simulink model "MMR_IntegratedSimulation_FUZZYTEST"  (R2013a)
settings: Solver=ode3  StartTime=0.0  StopTime=Tstop  FixedStep=1e-2  RelTol=1e-3
values from neighbouring files (symbols this model uses):
  B = 0.0141    [parameters.m]
  Experiment = 2    [parameters.m]
  J = 0.0294    [parameters.m]
  Ke = 0.65    [parameters.m]
  Kt = 0.65    [parameters.m]
  L = 0.04    [parameters.m]
  Len = dis    (= 0)    [calc_len.m]    (also in parameters.m = 0.2)
  r = round(t/step + 1)    [TrajGen_MMR_FUZZYTEST.m]    (also in parameters.m = 0.045)
  R = 3.07    [parameters.m]
  R1_phi = 0.0    (= 0)    [parameters.m]
  R1_xi = 2.0    (= 2)    [parameters.m]
  R1_yi = 0.9    [parameters.m]
  R2_phi = 0.0    (= 0)    [parameters.m]
  R2_xi = -1.0    (= -1)    [parameters.m]
  R2_yi = 4.0    (= 4)    [parameters.m]
  R3_phi = 0.0    (= 0)    [parameters.m]
  R3_xi = 2.0    (= 2)    [parameters.m]
  R3_yi = -1.2    [parameters.m]
  Tstop = 210    [parameters.m]
libraries: simulink x9, fuzblock x6, dsparch4 x3
(part 1 of 2)
settings Model: Creator=Hussain  LastModifiedBy=Hussain Aftab
settings DataIOCC: SignalLoggingSaveFormat=ModelDataLogs
settings DebuggingCC: FcnCallInpInsideContextMsg=EnableAllAsWarning
settings GRTTargetCC: CombineOutputUpdateFcns=off  GRTInterface=on

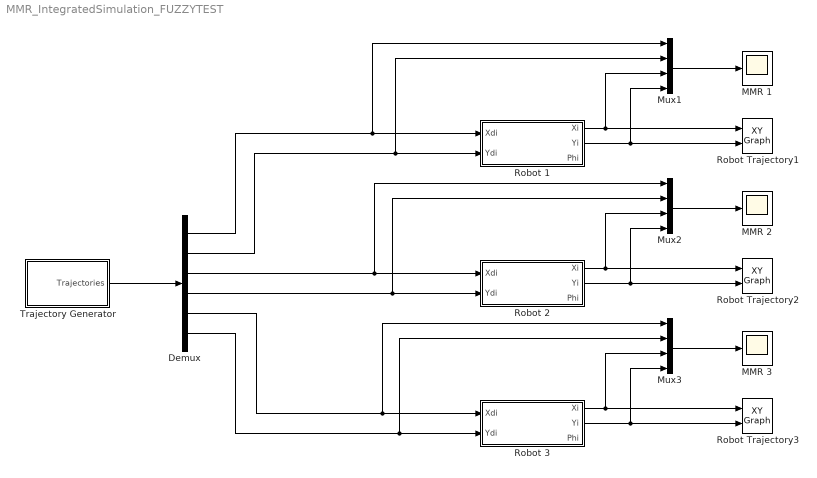
== system MMR_IntegratedSimulation_FUZZYTEST ==
  Demux : Demux  Outputs=6
  MMR 1 : Scope
      settings: TimeRange=100  YMin=0  YMax=10.5  SaveName=Robot1
  MMR 2 : Scope
      settings: TimeRange=100  YMin=0  YMax=10.5  SaveName=Robot2
  MMR 3 : Scope
      settings: TimeRange=100  YMin=0  YMax=10.5  SaveName=Robot3
  Mux1 : Mux
  Mux2 : Mux
  Mux3 : Mux
  Robot 1 : Subsystem
  Robot 2 : Subsystem
  Robot 3 : Subsystem
  Robot Trajectory1 : simulink/Sinks/XY Graph  xmin=0  xmax=15  ymin=-15  ymax=15  st=-1
  Robot Trajectory2 : simulink/Sinks/XY Graph  xmin=0  xmax=15  ymin=-15  ymax=15  st=-1
  Robot Trajectory3 : simulink/Sinks/XY Graph  xmin=0  xmax=15  ymin=-15  ymax=15  st=-1
  Trajectory Generator : Subsystem
  wires:
  Robot 1/1(Xi) -> Mux1/3, Robot Trajectory1/1
  Robot 1/2(Yi) -> Mux1/4, Robot Trajectory1/2
  Mux1/1 -> MMR 1/1
  Demux/4 -> Robot 2/2(Ydi), Mux2/2
  Demux/3 -> Mux2/1, Robot 2/1(Xdi)
  Robot 2/1(Xi) -> Mux2/3, Robot Trajectory2/1
  Robot 2/2(Yi) -> Mux2/4, Robot Trajectory2/2
  Mux2/1 -> MMR 2/1
  Demux/6 -> Mux3/2, Robot 3/2(Ydi)
  Demux/5 -> Mux3/1, Robot 3/1(Xdi)
  Robot 3/1(Xi) -> Mux3/3, Robot Trajectory3/1
  Robot 3/2(Yi) -> Mux3/4, Robot Trajectory3/2
  Mux3/1 -> MMR 3/1
  Demux/1 -> Mux1/1, Robot 1/1(Xdi)
  Demux/2 -> Mux1/2, Robot 1/2(Ydi)
  Trajectory Generator/1(Trajectories) -> Demux/1

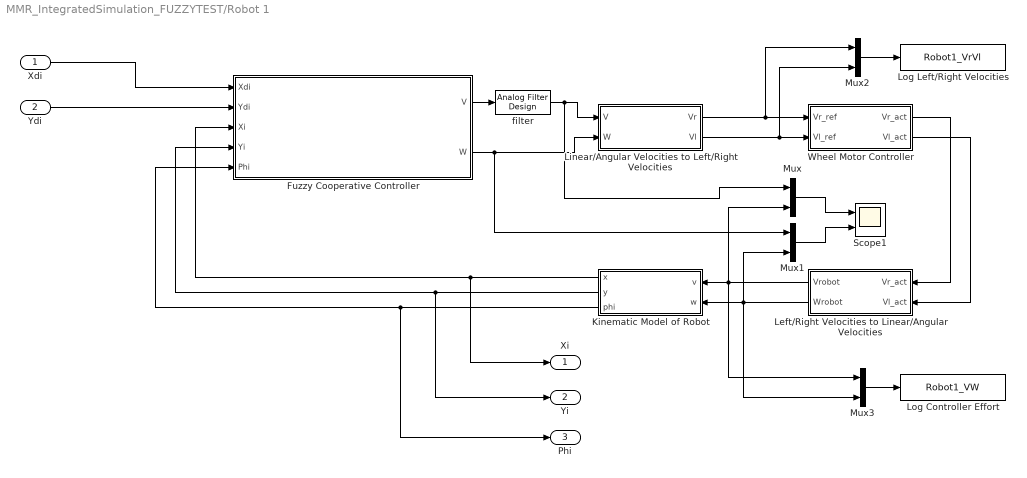
== system MMR_IntegratedSimulation_FUZZYTEST/Robot 1 ==
  Xdi : Inport
  Ydi : Inport  Port=2
  Fuzzy Cooperative Controller : Subsystem
  Kinematic Model of Robot : Subsystem
  Left/Right Velocities to Linear/Angular Velocities : Subsystem
  Linear/Angular Velocities to Left/Right Velocities : Subsystem
  Log Controller Effort : ToWorkspace  VariableName=Robot1_VW  SampleTime=-1  SaveFormat=Structure With Time
  Log Left/Right Velocities : ToWorkspace  VariableName=Robot1_VrVl  SampleTime=-1  SaveFormat=Structure With Time
  Mux{,1..3} (4 alike) : Mux  Inputs=2
  Scope1 : Scope  NumInputPorts=2
      settings: YMin=-5~-5  YMax=5~5  SaveName=ScopeData5
  Wheel Motor Controller : Subsystem
  filter : dsparch4/Analog Filter Design  method=Butterworth  filttype=Lowpass  N=5  Wlo=10  Whi=80  Rp=2  Rs=40
  Xi : Outport
  Yi : Outport  Port=2
  Phi : Outport  Port=3
  wires:
  Linear/Angular Velocities to Left/Right Velocities/1(Vr) -> Mux2/1, Wheel Motor Controller/1(Vr_ref)
  Linear/Angular Velocities to Left/Right Velocities/2(Vl) -> Mux2/2, Wheel Motor Controller/2(Vl_ref)
  Wheel Motor Controller/1(Vr_act) -> Left/Right Velocities to Linear/Angular Velocities/1(Vr_act)
  Wheel Motor Controller/2(Vl_act) -> Left/Right Velocities to Linear/Angular Velocities/2(Vl_act)
  Left/Right Velocities to Linear/Angular Velocities/1(Vrobot) -> Mux3/1, Mux/2, Kinematic Model of Robot/1(v)
  Left/Right Velocities to Linear/Angular Velocities/2(Wrobot) -> Mux3/2, Mux1/2, Kinematic Model of Robot/2(w)
  Fuzzy Cooperative Controller/2(W) -> Mux1/1, Linear/Angular Velocities to Left/Right Velocities/2(W)
  Xdi/1 -> Fuzzy Cooperative Controller/1(Xdi)
  Ydi/1 -> Fuzzy Cooperative Controller/2(Ydi)
  Kinematic Model of Robot/1(x) -> Fuzzy Cooperative Controller/3(Xi), Xi/1
  Kinematic Model of Robot/2(y) -> Fuzzy Cooperative Controller/4(Yi), Yi/1
  Kinematic Model of Robot/3(phi) -> Fuzzy Cooperative Controller/5(Phi), Phi/1
  Mux/1 -> Scope1/1
  Mux1/1 -> Scope1/2
  Mux2/1 -> Log Left/Right Velocities/1
  Mux3/1 -> Log Controller Effort/1
  filter/1 -> Mux/1, Linear/Angular Velocities to Left/Right Velocities/1(V)
  Fuzzy Cooperative Controller/1(V) -> filter/1

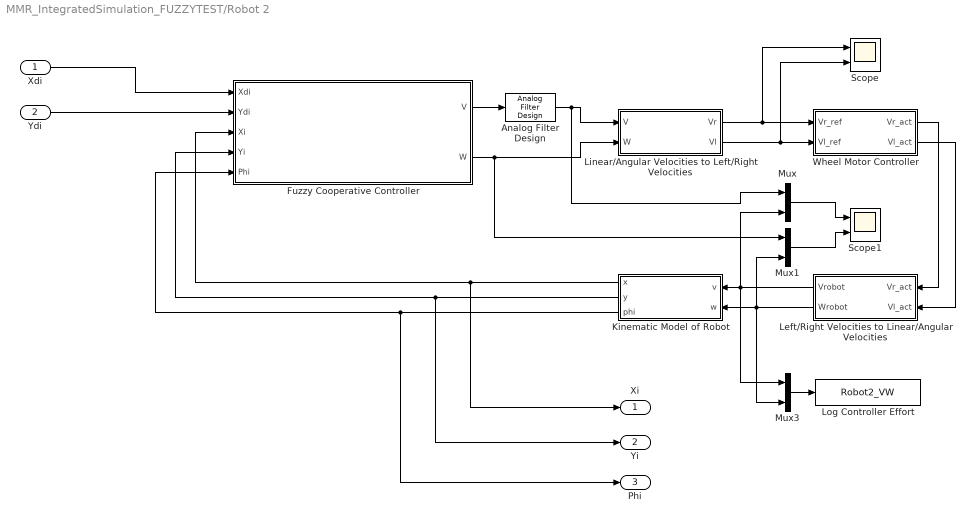
== system MMR_IntegratedSimulation_FUZZYTEST/Robot 2 ==
  Xdi : Inport
  Ydi : Inport  Port=2
  Analog Filter Design : dsparch4/Analog Filter Design  method=Butterworth  filttype=Lowpass  N=5  Wlo=10  Whi=80  Rp=2  Rs=40
  Fuzzy Cooperative Controller : Subsystem
  Kinematic Model of Robot : Subsystem
  Left/Right Velocities to Linear/Angular Velocities : Subsystem
  Linear/Angular Velocities to Left/Right Velocities : Subsystem
  Log Controller Effort : ToWorkspace  VariableName=Robot2_VW  SampleTime=-1  SaveFormat=Structure With Time
  Mux : Mux  Inputs=2
  Mux1 : Mux  Inputs=2
  Mux3 : Mux  Inputs=2
  Scope : Scope  NumInputPorts=2
      settings: YMin=-5~-5  YMax=5~5  SaveName=ScopeData3
  Scope1 : Scope  NumInputPorts=2
      settings: TimeRange=210  YMin=-5~-5  YMax=5~5  SaveName=ScopeData5
  Wheel Motor Controller : Subsystem
  Xi : Outport
  Yi : Outport  Port=2
  Phi : Outport  Port=3
  wires:
  Linear/Angular Velocities to Left/Right Velocities/1(Vr) -> Scope/1, Wheel Motor Controller/1(Vr_ref)
  Linear/Angular Velocities to Left/Right Velocities/2(Vl) -> Scope/2, Wheel Motor Controller/2(Vl_ref)
  Wheel Motor Controller/1(Vr_act) -> Left/Right Velocities to Linear/Angular Velocities/1(Vr_act)
  Wheel Motor Controller/2(Vl_act) -> Left/Right Velocities to Linear/Angular Velocities/2(Vl_act)
  Left/Right Velocities to Linear/Angular Velocities/1(Vrobot) -> Mux3/1, Mux/2, Kinematic Model of Robot/1(v)
  Left/Right Velocities to Linear/Angular Velocities/2(Wrobot) -> Mux3/2, Mux1/2, Kinematic Model of Robot/2(w)
  Xdi/1 -> Fuzzy Cooperative Controller/1(Xdi)
  Ydi/1 -> Fuzzy Cooperative Controller/2(Ydi)
  Kinematic Model of Robot/1(x) -> Fuzzy Cooperative Controller/3(Xi), Xi/1
  Kinematic Model of Robot/2(y) -> Fuzzy Cooperative Controller/4(Yi), Yi/1
  Kinematic Model of Robot/3(phi) -> Fuzzy Cooperative Controller/5(Phi), Phi/1
  Mux/1 -> Scope1/1
  Mux1/1 -> Scope1/2
  Fuzzy Cooperative Controller/2(W) -> Mux1/1, Linear/Angular Velocities to Left/Right Velocities/2(W)
  Mux3/1 -> Log Controller Effort/1
  Fuzzy Cooperative Controller/1(V) -> Analog Filter Design/1
  Analog Filter Design/1 -> Mux/1, Linear/Angular Velocities to Left/Right Velocities/1(V)

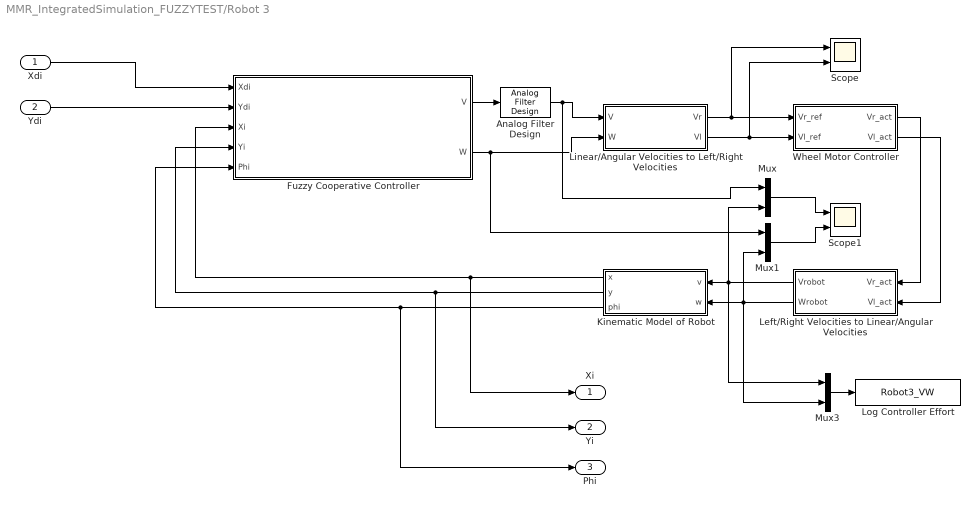
== system MMR_IntegratedSimulation_FUZZYTEST/Robot 3 ==
  Xdi : Inport
  Ydi : Inport  Port=2
  Analog Filter Design : dsparch4/Analog Filter Design  method=Butterworth  filttype=Lowpass  N=5  Wlo=10  Whi=80  Rp=2  Rs=40
  Fuzzy Cooperative Controller : Subsystem
  Kinematic Model of Robot : Subsystem
  Left/Right Velocities to Linear/Angular Velocities : Subsystem
  Linear/Angular Velocities to Left/Right Velocities : Subsystem
  Log Controller Effort : ToWorkspace  VariableName=Robot3_VW  SampleTime=-1  SaveFormat=Structure With Time
  Mux : Mux  Inputs=2
  Mux1 : Mux  Inputs=2
  Mux3 : Mux  Inputs=2
  Scope : Scope  NumInputPorts=2
      settings: YMin=-5~-5  YMax=5~5  SaveName=ScopeData3
  Scope1 : Scope  NumInputPorts=2
      settings: YMin=-5~-5  YMax=5~5  SaveName=ScopeData5
  Wheel Motor Controller : Subsystem
  Xi : Outport
  Yi : Outport  Port=2
  Phi : Outport  Port=3
  wires:
  Linear/Angular Velocities to Left/Right Velocities/1(Vr) -> Wheel Motor Controller/1(Vr_ref), Scope/1
  Linear/Angular Velocities to Left/Right Velocities/2(Vl) -> Wheel Motor Controller/2(Vl_ref), Scope/2
  Wheel Motor Controller/1(Vr_act) -> Left/Right Velocities to Linear/Angular Velocities/1(Vr_act)
  Wheel Motor Controller/2(Vl_act) -> Left/Right Velocities to Linear/Angular Velocities/2(Vl_act)
  Left/Right Velocities to Linear/Angular Velocities/1(Vrobot) -> Mux3/1, Mux/2, Kinematic Model of Robot/1(v)
  Left/Right Velocities to Linear/Angular Velocities/2(Wrobot) -> Mux3/2, Mux1/2, Kinematic Model of Robot/2(w)
  Xdi/1 -> Fuzzy Cooperative Controller/1(Xdi)
  Ydi/1 -> Fuzzy Cooperative Controller/2(Ydi)
  Kinematic Model of Robot/1(x) -> Fuzzy Cooperative Controller/3(Xi), Xi/1
  Kinematic Model of Robot/2(y) -> Fuzzy Cooperative Controller/4(Yi), Yi/1
  Kinematic Model of Robot/3(phi) -> Fuzzy Cooperative Controller/5(Phi), Phi/1
  Mux/1 -> Scope1/1
  Mux1/1 -> Scope1/2
  Fuzzy Cooperative Controller/2(W) -> Linear/Angular Velocities to Left/Right Velocities/2(W), Mux1/1
  Mux3/1 -> Log Controller Effort/1
  Fuzzy Cooperative Controller/1(V) -> Analog Filter Design/1
  Analog Filter Design/1 -> Mux/1, Linear/Angular Velocities to Left/Right Velocities/1(V)

== system MMR_IntegratedSimulation_FUZZYTEST/Trajectory Generator ==
  Experiment # : Constant  Value=Experiment
  Mux2 : Mux  Inputs=3
  Simulation Time : Clock
  Stop Time : Constant  Value=Tstop
  Trajectory Generation Function : MATLABFcn  MATLABFcn=TrajGen_MMR_FUZZYTEST
  Trajectories : Outport
  wires:
  Simulation Time/1 -> Mux2/1
  Trajectory Generation Function/1 -> Trajectories/1
  Mux2/1 -> Trajectory Generation Function/1
  Stop Time/1 -> Mux2/2
  Experiment #/1 -> Mux2/3

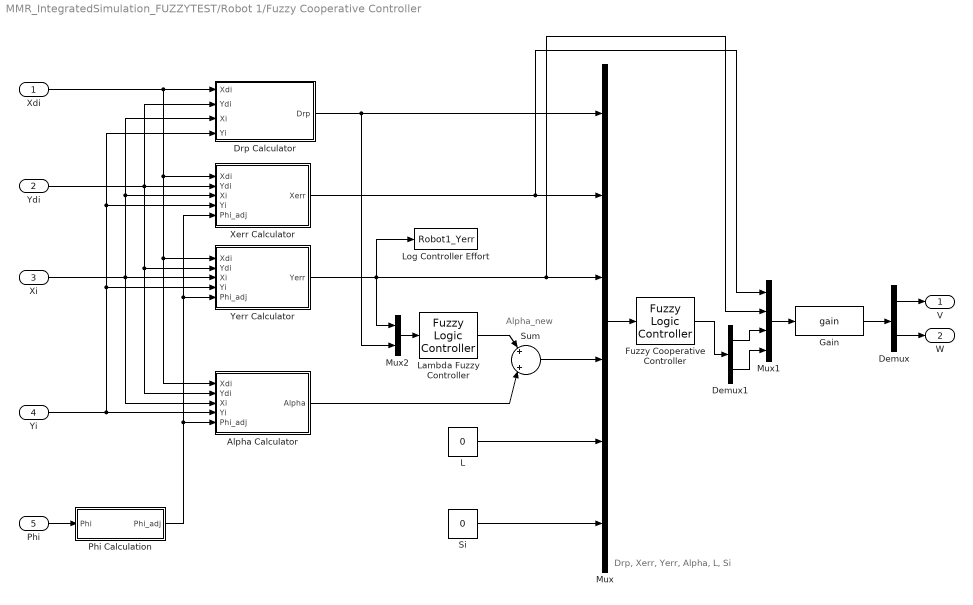
== system MMR_IntegratedSimulation_FUZZYTEST/Robot 1/Fuzzy Cooperative Controller ==
  note: Alpha_new
  note: Drp, Xerr, Yerr, Alpha, L, Si
  Xdi : Inport
  Ydi : Inport  Port=2
  Xi : Inport  Port=3
  Yi : Inport  Port=4
  Phi : Inport  Port=5
  Alpha Calculator : Subsystem
  Demux : Demux  Outputs=2
  Demux1 : Demux  Outputs=2
  Drp Calculator : Subsystem
  Fuzzy Cooperative Controller : fuzblock/Fuzzy Logic  Controller  fis=FuzzyCoperativeController
  Gain : MATLABFcn  MATLABFcn=gain
  L : Constant  Value=0
  Lambda Fuzzy Controller : fuzblock/Fuzzy Logic  Controller  fis=LamdaFuzzyController
  Log Controller Effort : ToWorkspace  VariableName=Robot1_Yerr  SampleTime=-1  SaveFormat=Structure With Time
  Mux : Mux  Inputs=6
  Mux1 : Mux
  Mux2 : Mux  Inputs=2
  Phi Calculation : Subsystem
  Si : Constant  Value=0
  Sum : Sum  Inputs=|+||+|
  Xerr Calculator : Subsystem
  Yerr Calculator : Subsystem
  V : Outport
  W : Outport  Port=2
  wires:
  Mux/1 -> Fuzzy Cooperative Controller/1
  Xerr Calculator/1(Xerr) -> Mux1/1, Mux/2
  L/1 -> Mux/5
  Si/1 -> Mux/6
  Sum/1 -> Mux/4
  Alpha Calculator/1(Alpha) -> Sum/2
  Yerr Calculator/1(Yerr) -> Mux1/2, Mux/3, Log Controller Effort/1, Mux2/1
  Drp Calculator/1(Drp) -> Mux2/2, Mux/1
  Lambda Fuzzy Controller/1 -> Sum/1
  Mux2/1 -> Lambda Fuzzy Controller/1
  Xdi/1 -> Drp Calculator/1(Xdi), Xerr Calculator/1(Xdi), Yerr Calculator/1(Xdi), Alpha Calculator/1(Xdi)
  Ydi/1 -> Xerr Calculator/2(Ydi), Drp Calculator/2(Ydi), Yerr Calculator/2(Ydi), Alpha Calculator/2(Ydi)
  Xi/1 -> Yerr Calculator/3(Xi), Drp Calculator/3(Xi), Xerr Calculator/3(Xi), Alpha Calculator/3(Xi)
  Yi/1 -> Alpha Calculator/4(Yi), Drp Calculator/4(Yi), Xerr Calculator/4(Yi), Yerr Calculator/4(Yi)
  Phi/1 -> Phi Calculation/1(Phi)
  Phi Calculation/1(Phi_adj) -> Yerr Calculator/5(Phi_adj), Xerr Calculator/5(Phi_adj), Alpha Calculator/5(Phi_adj)
  Demux/1 -> V/1
  Demux/2 -> W/1
  Mux1/1 -> Gain/1
  Gain/1 -> Demux/1
  Demux1/1 -> Mux1/3
  Demux1/2 -> Mux1/4
  Fuzzy Cooperative Controller/1 -> Demux1/1

== system MMR_IntegratedSimulation_FUZZYTEST/Robot 1/Kinematic Model of Robot ==
  note: phi_dot
  note: y_dot
  note: x_dot
  note: phi
  note: y
  note: x
  v : Inport
  w : Inport  Port=2
  Fcn : Fcn  Expr=cos(u)
  Fcn1 : Fcn  Expr=sin(u)
  Integrator : Integrator  InitialCondition=R1_xi
  Integrator1 : Integrator  InitialCondition=R1_yi
  Integrator2 : Integrator  InitialCondition=R1_phi
  Product : Product
  Product1 : Product
  x : Outport
  y : Outport  Port=2
  phi : Outport  Port=3
  wires:
  Product1/1 -> Integrator1/1
  Integrator/1 -> x/1
  Integrator1/1 -> y/1
  v/1 -> Product1/1, Product/1
  Product/1 -> Integrator/1
  Fcn/1 -> Product/2
  Fcn1/1 -> Product1/2
  Integrator2/1 -> Fcn/1, Fcn1/1, phi/1
  w/1 -> Integrator2/1

== system MMR_IntegratedSimulation_FUZZYTEST/Robot 1/Left//Right Velocities to Linear//Angular Velocities ==
  Vr_act : Inport
  Vl_act : Inport  Port=2
  Calculate Vrobot : Fcn  Expr="(  u(1) + u(2) ) / 2"
  Calculate Wrobot : Fcn  Expr="(  u(1) - u(2) ) / Len"
  Mux : Mux  Inputs=2
  Vrobot : Outport
  Wrobot : Outport  Port=2
  wires:
  Vr_act/1 -> Mux/1
  Vl_act/1 -> Mux/2
  Mux/1 -> Calculate Vrobot/1, Calculate Wrobot/1
  Calculate Vrobot/1 -> Vrobot/1
  Calculate Wrobot/1 -> Wrobot/1

== system MMR_IntegratedSimulation_FUZZYTEST/Robot 1/Linear//Angular Velocities to Left//Right Velocities ==
  V : Inport
  W : Inport  Port=2
  Calculate Vl : Fcn  Expr=( 2 * u(1) - u(2) * Len ) / 2
  Calculate Vr : Fcn  Expr=( 2 * u(1) + u(2) * Len ) / 2
  Mux : Mux  Inputs=2
  Vr : Outport
  Vl : Outport  Port=2
  wires:
  V/1 -> Mux/1
  W/1 -> Mux/2
  Mux/1 -> Calculate Vr/1, Calculate Vl/1
  Calculate Vr/1 -> Vr/1
  Calculate Vl/1 -> Vl/1

== system MMR_IntegratedSimulation_FUZZYTEST/Robot 1/Wheel Motor Controller ==
  note: Linear to Angular Velocity Conversion
  note: Wl
  note: Wr
  note: Linear to Angular Velocity Conversion
  note: Angular to Linear Velocity Conversion
  note: Angular to Linear Velocity Conversion
  Vr_ref : Inport
  Vl_ref : Inport  Port=2
  Gain : Gain  Gain=1/r
  Gain1 : Gain  Gain=1/r
  Gain2 : Gain  Gain=r
  Gain3 : Gain  Gain=r
  Left Motor Speed Controller and Motor Model : Subsystem
  Right Motor Speed Controller and Motor Model : Subsystem
  Vr_act : Outport
  Vl_act : Outport  Port=2
  wires:
  Vl_ref/1 -> Gain1/1
  Vr_ref/1 -> Gain/1
  Gain/1 -> Right Motor Speed Controller and Motor Model/1(W_ref)
  Gain1/1 -> Left Motor Speed Controller and Motor Model/1(W_ref)
  Left Motor Speed Controller and Motor Model/1(W_act) -> Gain3/1
  Gain3/1 -> Vl_act/1
  Right Motor Speed Controller and Motor Model/1(W_act) -> Gain2/1
  Gain2/1 -> Vr_act/1

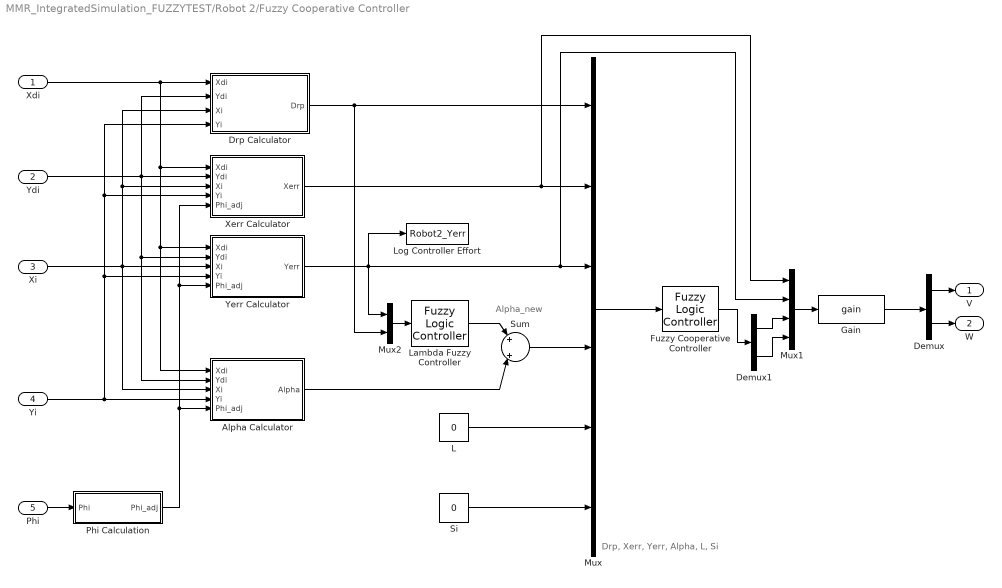
== system MMR_IntegratedSimulation_FUZZYTEST/Robot 2/Fuzzy Cooperative Controller ==
  note: Alpha_new
  note: Drp, Xerr, Yerr, Alpha, L, Si
  Xdi : Inport
  Ydi : Inport  Port=2
  Xi : Inport  Port=3
  Yi : Inport  Port=4
  Phi : Inport  Port=5
  Alpha Calculator : Subsystem
  Demux : Demux  Outputs=2
  Demux1 : Demux  Outputs=2
  Drp Calculator : Subsystem
  Fuzzy Cooperative Controller : fuzblock/Fuzzy Logic  Controller  fis=FuzzyCoperativeController
  Gain : MATLABFcn  MATLABFcn=gain
  L : Constant  Value=0
  Lambda Fuzzy Controller : fuzblock/Fuzzy Logic  Controller  fis=LamdaFuzzyController
  Log Controller Effort : ToWorkspace  VariableName=Robot2_Yerr  SampleTime=-1  SaveFormat=Structure With Time
  Mux : Mux  Inputs=6
  Mux1 : Mux
  Mux2 : Mux  Inputs=2
  Phi Calculation : Subsystem
  Si : Constant  Value=0
  Sum : Sum  Inputs=|+||+|
  Xerr Calculator : Subsystem
  Yerr Calculator : Subsystem
  V : Outport
  W : Outport  Port=2
  wires:
  Mux/1 -> Fuzzy Cooperative Controller/1
  Xerr Calculator/1(Xerr) -> Mux1/1, Mux/2
  L/1 -> Mux/5
  Si/1 -> Mux/6
  Sum/1 -> Mux/4
  Alpha Calculator/1(Alpha) -> Sum/2
  Yerr Calculator/1(Yerr) -> Log Controller Effort/1, Mux2/1, Mux1/2, Mux/3
  Drp Calculator/1(Drp) -> Mux2/2, Mux/1
  Lambda Fuzzy Controller/1 -> Sum/1
  Mux2/1 -> Lambda Fuzzy Controller/1
  Xdi/1 -> Drp Calculator/1(Xdi), Xerr Calculator/1(Xdi), Yerr Calculator/1(Xdi), Alpha Calculator/1(Xdi)
  Ydi/1 -> Xerr Calculator/2(Ydi), Drp Calculator/2(Ydi), Yerr Calculator/2(Ydi), Alpha Calculator/2(Ydi)
  Xi/1 -> Yerr Calculator/3(Xi), Drp Calculator/3(Xi), Xerr Calculator/3(Xi), Alpha Calculator/3(Xi)
  Yi/1 -> Alpha Calculator/4(Yi), Drp Calculator/4(Yi), Xerr Calculator/4(Yi), Yerr Calculator/4(Yi)
  Phi/1 -> Phi Calculation/1(Phi)
  Phi Calculation/1(Phi_adj) -> Yerr Calculator/5(Phi_adj), Xerr Calculator/5(Phi_adj), Alpha Calculator/5(Phi_adj)
  Demux/1 -> V/1
  Demux/2 -> W/1
  Mux1/1 -> Gain/1
  Demux1/1 -> Mux1/3
  Demux1/2 -> Mux1/4
  Fuzzy Cooperative Controller/1 -> Demux1/1
  Gain/1 -> Demux/1

== system MMR_IntegratedSimulation_FUZZYTEST/Robot 2/Kinematic Model of Robot ==
  note: phi_dot
  note: y_dot
  note: x_dot
  note: phi
  note: y
  note: x
  v : Inport
  w : Inport  Port=2
  Fcn : Fcn  Expr=cos(u)
  Fcn1 : Fcn  Expr=sin(u)
  Integrator : Integrator  InitialCondition=R2_xi
  Integrator1 : Integrator  InitialCondition=R2_yi
  Integrator2 : Integrator  InitialCondition=R2_phi
  Product : Product
  Product1 : Product
  x : Outport
  y : Outport  Port=2
  phi : Outport  Port=3
  wires:
  Product1/1 -> Integrator1/1
  Integrator/1 -> x/1
  Integrator1/1 -> y/1
  v/1 -> Product1/1, Product/1
  Product/1 -> Integrator/1
  Fcn/1 -> Product/2
  Fcn1/1 -> Product1/2
  Integrator2/1 -> Fcn/1, Fcn1/1, phi/1
  w/1 -> Integrator2/1

== system MMR_IntegratedSimulation_FUZZYTEST/Robot 2/Left//Right Velocities to Linear//Angular Velocities ==
  Vr_act : Inport
  Vl_act : Inport  Port=2
  Calculate Vrobot : Fcn  Expr="(  u(1) + u(2) ) / 2"
  Calculate Wrobot : Fcn  Expr="(  u(1) - u(2) ) / Len"
  Mux : Mux  Inputs=2
  Vrobot : Outport
  Wrobot : Outport  Port=2
  wires:
  Vr_act/1 -> Mux/1
  Vl_act/1 -> Mux/2
  Mux/1 -> Calculate Vrobot/1, Calculate Wrobot/1
  Calculate Vrobot/1 -> Vrobot/1
  Calculate Wrobot/1 -> Wrobot/1

== system MMR_IntegratedSimulation_FUZZYTEST/Robot 2/Linear//Angular Velocities to Left//Right Velocities ==
  V : Inport
  W : Inport  Port=2
  Calculate Vl : Fcn  Expr=( 2 * u(1) - u(2) * Len ) / 2
  Calculate Vr : Fcn  Expr=( 2 * u(1) + u(2) * Len ) / 2
  Mux : Mux  Inputs=2
  Vr : Outport
  Vl : Outport  Port=2
  wires:
  V/1 -> Mux/1
  W/1 -> Mux/2
  Mux/1 -> Calculate Vr/1, Calculate Vl/1
  Calculate Vr/1 -> Vr/1
  Calculate Vl/1 -> Vl/1

== system MMR_IntegratedSimulation_FUZZYTEST/Robot 2/Wheel Motor Controller ==
  note: Linear to Angular Velocity Conversion
  note: Wl
  note: Wr
  note: Linear to Angular Velocity Conversion
  note: Angular to Linear Velocity Conversion
  note: Angular to Linear Velocity Conversion
  Vr_ref : Inport
  Vl_ref : Inport  Port=2
  Gain : Gain  Gain=1/r
  Gain1 : Gain  Gain=1/r
  Gain2 : Gain  Gain=r
  Gain3 : Gain  Gain=r
  Left Motor Speed Controller and Motor Model : Subsystem
  Right Motor Speed Controller and Motor Model : Subsystem
  Vr_act : Outport
  Vl_act : Outport  Port=2
  wires:
  Vl_ref/1 -> Gain1/1
  Vr_ref/1 -> Gain/1
  Gain/1 -> Right Motor Speed Controller and Motor Model/1(W_ref)
  Gain1/1 -> Left Motor Speed Controller and Motor Model/1(W_ref)
  Left Motor Speed Controller and Motor Model/1(W_act) -> Gain3/1
  Gain3/1 -> Vl_act/1
  Right Motor Speed Controller and Motor Model/1(W_act) -> Gain2/1
  Gain2/1 -> Vr_act/1

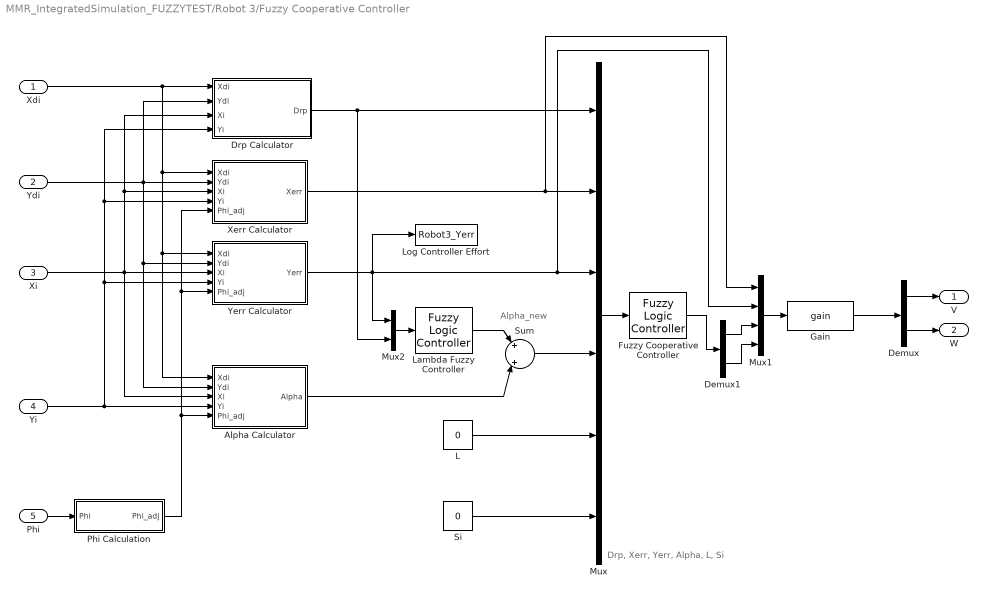
== system MMR_IntegratedSimulation_FUZZYTEST/Robot 3/Fuzzy Cooperative Controller ==
  note: Alpha_new
  note: Drp, Xerr, Yerr, Alpha, L, Si
  Xdi : Inport
  Ydi : Inport  Port=2
  Xi : Inport  Port=3
  Yi : Inport  Port=4
  Phi : Inport  Port=5
  Alpha Calculator : Subsystem
  Demux : Demux  Outputs=2
  Demux1 : Demux  Outputs=2
  Drp Calculator : Subsystem
  Fuzzy Cooperative Controller : fuzblock/Fuzzy Logic  Controller  fis=FuzzyCoperativeController
  Gain : MATLABFcn  MATLABFcn=gain
  L : Constant  Value=0
  Lambda Fuzzy Controller : fuzblock/Fuzzy Logic  Controller  fis=LamdaFuzzyController
  Log Controller Effort : ToWorkspace  VariableName=Robot3_Yerr  SampleTime=-1  SaveFormat=Structure With Time
  Mux : Mux  Inputs=6
  Mux1 : Mux
  Mux2 : Mux  Inputs=2
  Phi Calculation : Subsystem
  Si : Constant  Value=0
  Sum : Sum  Inputs=|+||+|
  Xerr Calculator : Subsystem
  Yerr Calculator : Subsystem
  V : Outport
  W : Outport  Port=2
  wires:
  Mux/1 -> Fuzzy Cooperative Controller/1
  Xerr Calculator/1(Xerr) -> Mux1/1, Mux/2
  L/1 -> Mux/5
  Si/1 -> Mux/6
  Sum/1 -> Mux/4
  Alpha Calculator/1(Alpha) -> Sum/2
  Yerr Calculator/1(Yerr) -> Log Controller Effort/1, Mux2/1, Mux1/2, Mux/3
  Drp Calculator/1(Drp) -> Mux2/2, Mux/1
  Lambda Fuzzy Controller/1 -> Sum/1
  Mux2/1 -> Lambda Fuzzy Controller/1
  Xdi/1 -> Drp Calculator/1(Xdi), Xerr Calculator/1(Xdi), Yerr Calculator/1(Xdi), Alpha Calculator/1(Xdi)
  Ydi/1 -> Xerr Calculator/2(Ydi), Drp Calculator/2(Ydi), Yerr Calculator/2(Ydi), Alpha Calculator/2(Ydi)
  Xi/1 -> Yerr Calculator/3(Xi), Drp Calculator/3(Xi), Xerr Calculator/3(Xi), Alpha Calculator/3(Xi)
  Yi/1 -> Alpha Calculator/4(Yi), Drp Calculator/4(Yi), Xerr Calculator/4(Yi), Yerr Calculator/4(Yi)
  Phi/1 -> Phi Calculation/1(Phi)
  Phi Calculation/1(Phi_adj) -> Yerr Calculator/5(Phi_adj), Xerr Calculator/5(Phi_adj), Alpha Calculator/5(Phi_adj)
  Demux/1 -> V/1
  Demux/2 -> W/1
  Mux1/1 -> Gain/1
  Demux1/1 -> Mux1/3
  Demux1/2 -> Mux1/4
  Fuzzy Cooperative Controller/1 -> Demux1/1
  Gain/1 -> Demux/1

== system MMR_IntegratedSimulation_FUZZYTEST/Robot 3/Kinematic Model of Robot ==
  note: phi_dot
  note: y_dot
  note: x_dot
  note: phi
  note: y
  note: x
  v : Inport
  w : Inport  Port=2
  Fcn : Fcn  Expr=cos(u)
  Fcn1 : Fcn  Expr=sin(u)
  Integrator : Integrator  InitialCondition=R3_xi
  Integrator1 : Integrator  InitialCondition=R3_yi
  Integrator2 : Integrator  InitialCondition=R3_phi
  Product : Product
  Product1 : Product
  x : Outport
  y : Outport  Port=2
  phi : Outport  Port=3
  wires:
  Product1/1 -> Integrator1/1
  Integrator/1 -> x/1
  Integrator1/1 -> y/1
  v/1 -> Product1/1, Product/1
  Product/1 -> Integrator/1
  Fcn/1 -> Product/2
  Fcn1/1 -> Product1/2
  Integrator2/1 -> Fcn/1, Fcn1/1, phi/1
  w/1 -> Integrator2/1

== system MMR_IntegratedSimulation_FUZZYTEST/Robot 3/Left//Right Velocities to Linear//Angular Velocities ==
  Vr_act : Inport
  Vl_act : Inport  Port=2
  Calculate Vrobot : Fcn  Expr="(  u(1) + u(2) ) / 2"
  Calculate Wrobot : Fcn  Expr="(  u(1) - u(2) ) / Len"
  Mux : Mux  Inputs=2
  Vrobot : Outport
  Wrobot : Outport  Port=2
  wires:
  Vr_act/1 -> Mux/1
  Vl_act/1 -> Mux/2
  Mux/1 -> Calculate Vrobot/1, Calculate Wrobot/1
  Calculate Vrobot/1 -> Vrobot/1
  Calculate Wrobot/1 -> Wrobot/1

== system MMR_IntegratedSimulation_FUZZYTEST/Robot 3/Linear//Angular Velocities to Left//Right Velocities ==
  V : Inport
  W : Inport  Port=2
  Calculate Vl : Fcn  Expr=( 2 * u(1) - u(2) * Len ) / 2
  Calculate Vr : Fcn  Expr=( 2 * u(1) + u(2) * Len ) / 2
  Mux : Mux  Inputs=2
  Vr : Outport
  Vl : Outport  Port=2
  wires:
  V/1 -> Mux/1
  W/1 -> Mux/2
  Mux/1 -> Calculate Vr/1, Calculate Vl/1
  Calculate Vr/1 -> Vr/1
  Calculate Vl/1 -> Vl/1

== system MMR_IntegratedSimulation_FUZZYTEST/Robot 3/Wheel Motor Controller ==
  note: Linear to Angular Velocity Conversion
  note: Wl
  note: Wr
  note: Linear to Angular Velocity Conversion
  note: Angular to Linear Velocity Conversion
  note: Angular to Linear Velocity Conversion
  Vr_ref : Inport
  Vl_ref : Inport  Port=2
  Gain : Gain  Gain=1/r
  Gain1 : Gain  Gain=1/r
  Gain2 : Gain  Gain=r
  Gain3 : Gain  Gain=r
  Left Motor Speed Controller and Motor Model : Subsystem
  Right Motor Speed Controller and Motor Model : Subsystem
  Vr_act : Outport
  Vl_act : Outport  Port=2
  wires:
  Vl_ref/1 -> Gain1/1
  Vr_ref/1 -> Gain/1
  Gain/1 -> Right Motor Speed Controller and Motor Model/1(W_ref)
  Gain1/1 -> Left Motor Speed Controller and Motor Model/1(W_ref)
  Left Motor Speed Controller and Motor Model/1(W_act) -> Gain3/1
  Gain3/1 -> Vl_act/1
  Right Motor Speed Controller and Motor Model/1(W_act) -> Gain2/1
  Gain2/1 -> Vr_act/1

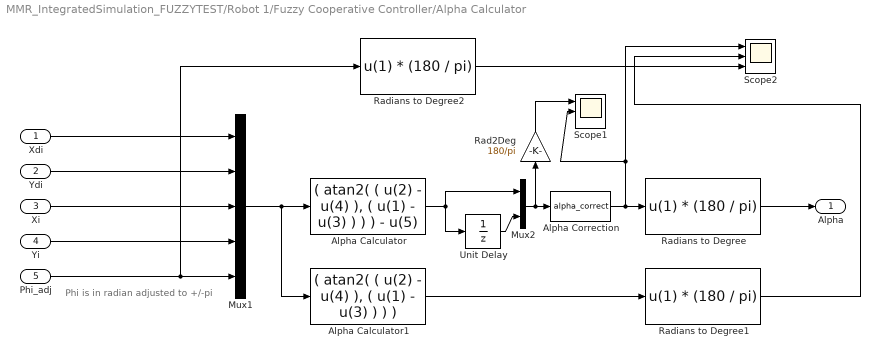
== system MMR_IntegratedSimulation_FUZZYTEST/Robot 1/Fuzzy Cooperative Controller/Alpha Calculator ==
  note: Phi is in radian adjusted to +/-pi
  Xdi : Inport
  Ydi : Inport  Port=2
  Xi : Inport  Port=3
  Yi : Inport  Port=4
  Phi_adj : Inport  Port=5
  Alpha Calculator : Fcn  Expr=( atan2( ( u(2) - u(4) ), ( u(1) - u(3) ) ) ) - u(5)
  Alpha Calculator1 : Fcn  Expr=( atan2( ( u(2) - u(4) ), ( u(1) - u(3) ) ) )
  Alpha Correction : MATLABFcn  MATLABFcn=alpha_correct
  Mux1 : Mux  Inputs=5
  Mux2 : Mux  Inputs=2
  Rad2Deg : Gain  Gain=180/pi
  Radians to Degree : Fcn  Expr=u(1) * (180 / pi)
  Radians to Degree1 : Fcn  Expr=u(1) * (180 / pi)
  Radians to Degree2 : Fcn  Expr=u(1) * (180 / pi)
  Scope1 : Scope  NumInputPorts=3
      settings: YMin=-325~-200~-175  YMax=50~200~200  SaveName=ScopeData4
  Scope2 : Scope  NumInputPorts=3
      settings: YMin=-325~-200~-175  YMax=50~200~200  SaveName=ScopeData2
  Unit Delay : UnitDelay  SampleTime=-1
  Alpha : Outport
  wires:
  Xi/1 -> Mux1/3
  Ydi/1 -> Mux1/2
  Xdi/1 -> Mux1/1
  Mux1/1 -> Alpha Calculator1/1, Alpha Calculator/1
  Yi/1 -> Mux1/4
  Phi_adj/1 -> Mux1/5, Radians to Degree2/1
  Radians to Degree/1 -> Alpha/1
  Alpha Calculator1/1 -> Radians to Degree1/1
  Radians to Degree1/1 -> Scope2/2
  Radians to Degree2/1 -> Scope2/3
  Alpha Correction/1 -> Radians to Degree/1, Scope2/1, Scope1/2
  Mux2/1 -> Alpha Correction/1, Rad2Deg/1
  Alpha Calculator/1 -> Unit Delay/1, Mux2/1
  Unit Delay/1 -> Mux2/2
  Rad2Deg/1 -> Scope1/1

== system MMR_IntegratedSimulation_FUZZYTEST/Robot 1/Fuzzy Cooperative Controller/Drp Calculator ==
  Xdi : Inport
  Ydi : Inport  Port=2
  Xi : Inport  Port=3
  Yi : Inport  Port=4
  Calculate Distance : Fcn  Expr="sqrt( ( u(1) - u(3) )^2 +  ( u(2) - u(4) )^2   )"
  Mux1 : Mux
  Drp : Outport
  wires:
  Mux1/1 -> Calculate Distance/1
  Calculate Distance/1 -> Drp/1
  Xdi/1 -> Mux1/1
  Ydi/1 -> Mux1/2
  Xi/1 -> Mux1/3
  Yi/1 -> Mux1/4

== system MMR_IntegratedSimulation_FUZZYTEST/Robot 1/Fuzzy Cooperative Controller/Phi Calculation ==
  Phi : Inport
  Interpreted MATLAB Function : MATLABFcn  MATLABFcn=PhiAdjust
  Phi_adj : Outport
  wires:
  Phi/1 -> Interpreted MATLAB Function/1
  Interpreted MATLAB Function/1 -> Phi_adj/1

== system MMR_IntegratedSimulation_FUZZYTEST/Robot 1/Fuzzy Cooperative Controller/Xerr Calculator ==
  note: Phi is in radian adjusted to +/-pi
  Xdi : Inport
  Ydi : Inport  Port=2
  Xi : Inport  Port=3
  Yi : Inport  Port=4
  Phi_adj : Inport  Port=5
  Mux1 : Mux  Inputs=5
  Xerr Distance : Fcn  Expr="( cos( u(5) ) * ( u(1) - u(3) ) ) +  ( sin( u(5) ) * ( ( u(2) - u(4) ) ) )"
  Xerr : Outport
  wires:
  Xi/1 -> Mux1/3
  Ydi/1 -> Mux1/2
  Xdi/1 -> Mux1/1
  Xerr Distance/1 -> Xerr/1
  Mux1/1 -> Xerr Distance/1
  Yi/1 -> Mux1/4
  Phi_adj/1 -> Mux1/5

== system MMR_IntegratedSimulation_FUZZYTEST/Robot 1/Fuzzy Cooperative Controller/Yerr Calculator ==
  note: Phi is in radian adjusted to +/-pi
  Xdi : Inport
  Ydi : Inport  Port=2
  Xi : Inport  Port=3
  Yi : Inport  Port=4
  Phi_adj : Inport  Port=5
  Mux1 : Mux  Inputs=5
  Yerr Distance : Fcn  Expr=-( sin( u(5) ) * ( ( u(1) - u(3) ) ) ) + ( cos( u(5) ) * ( u(2) - u(4) ) )
  Yerr : Outport
  wires:
  Phi_adj/1 -> Mux1/5
  Yi/1 -> Mux1/4
  Mux1/1 -> Yerr Distance/1
  Yerr Distance/1 -> Yerr/1
  Xdi/1 -> Mux1/1
  Ydi/1 -> Mux1/2
  Xi/1 -> Mux1/3

== system MMR_IntegratedSimulation_FUZZYTEST/Robot 1/Wheel Motor Controller/Left Motor Speed Controller and Motor Model ==
  W_ref : Inport
  Left Motor Ref vs Act Speed : Scope
      settings: TimeRange=20  YMin=-0.01  YMax=0.12  SaveName=ScopeData6
  Load Torque : Constant  Value=0
  Mux : Mux  Inputs=2
  PMDC Motor Model : Subsystem
  Quantizer : Quantizer  QuantizationInterval=0.001
  Right Motor : Scope  NumInputPorts=3
      settings: TimeRange=20  YMin=-5~-5~-5  YMax=5~5~5
  Saturation : Saturate  UpperLimit=2000  LowerLimit=-2000
  Speed PID Controller : simulink/Continuous/PID Controller  Controller=PID  TimeDomain=Continuous-time  SampleTime=1  IntegratorMethod=Forward Euler  FilterMethod=Forward Euler  Form=Parallel  P=1.39131822817714  I=9.69423314548269  D=-0.0516542631137251  N=13.2920819861493  InitialConditionSource=internal  InitialConditionForIntegrator=0  InitialConditionForFilter=0  ExternalReset=none  LimitOutput=off  UpperSaturationLimit=160  LowerSaturationLimit=-160  LinearizeAsGain=on  AntiWindupMode=none  Kb=1  TrackingMode=off  Kt=1  PParamMin=[]  PParamMax=[]  IParamMin=[]  IParamMax=[]  DParamMin=[]  DParamMax=[]  NParamMin=[]  NParamMax=[]  KbParamMin=[]  KbParamMax=[]  KtParamMin=[]  KtParamMax=[]  POutMin=[]  POutMax=[]  IOutMin=[]  IOutMax=[]  DOutMin=[]  DOutMax=[]  NOutMin=[]  NOutMax=[]  KbOutMin=[]  KbOutMax=[]  KtOutMin=[]  KtOutMax=[]  IntegratorOutMin=[]  IntegratorOutMax=[]  FilterOutMin=[]  FilterOutMax=[]  SumOutMin=[]  SumOutMax=[]  SumI1OutMin=[]  SumI1OutMax=[]  SumI2OutMin=[]  SumI2OutMax=[]  SumI3OutMin=[]  SumI3OutMax=[]  SumDOutMin=[]  SumDOutMax=[]  SaturationOutMin=[]  SaturationOutMax=[]  IntegratorContinuousStateAttributes=''  IntegratorStateMustResolveToSignalObject=off  IntegratorRTWStateStorageClass=Auto  FilterContinuousStateAttributes=''  FilterStateMustResolveToSignalObject=off  FilterRTWStateStorageClass=Auto
  Sum1 : Sum  Inputs=|+-
  W_act : Outport
  wires:
  Speed PID Controller/1 -> PMDC Motor Model/1(V)
  Saturation/1 -> Sum1/1
  PMDC Motor Model/2(w) -> Quantizer/1
  Sum1/1 -> Speed PID Controller/1
  PMDC Motor Model/3(I) -> Right Motor/3
  PMDC Motor Model/1(Theta) -> Right Motor/1
  W_ref/1 -> Mux/1, Saturation/1
  Load Torque/1 -> PMDC Motor Model/2(Tl)
  Mux/1 -> Left Motor Ref vs Act Speed/1
  Quantizer/1 -> W_act/1, Mux/2, Sum1/2, Right Motor/2

== system MMR_IntegratedSimulation_FUZZYTEST/Robot 1/Wheel Motor Controller/Right Motor Speed Controller and Motor Model ==
  W_ref : Inport
  Load Torque : Constant  Value=0
  Mux : Mux  Inputs=2
  PMDC Motor Model : Subsystem
  Quantizer : Quantizer  QuantizationInterval=0.001
  Right Motor : Scope  NumInputPorts=3
      settings: TimeRange=20  YMin=-5~-5~-5  YMax=5~5~5
  Right Motor Ref vs Act Speed : Scope
      settings: TimeRange=20  YMin=-0.01  YMax=0.12
  Saturation : Saturate  UpperLimit=209.4  LowerLimit=-2000
  Speed PID Controller : simulink/Continuous/PID Controller  Controller=PID  TimeDomain=Continuous-time  SampleTime=1  IntegratorMethod=Forward Euler  FilterMethod=Forward Euler  Form=Parallel  P=1.39131822817714  I=9.69423314548269  D=-0.0516542631137251  N=13.2920819861493  InitialConditionSource=internal  InitialConditionForIntegrator=0  InitialConditionForFilter=0  ExternalReset=none  LimitOutput=off  UpperSaturationLimit=160  LowerSaturationLimit=-160  LinearizeAsGain=on  AntiWindupMode=none  Kb=1  TrackingMode=off  Kt=1  PParamMin=[]  PParamMax=[]  IParamMin=[]  IParamMax=[]  DParamMin=[]  DParamMax=[]  NParamMin=[]  NParamMax=[]  KbParamMin=[]  KbParamMax=[]  KtParamMin=[]  KtParamMax=[]  POutMin=[]  POutMax=[]  IOutMin=[]  IOutMax=[]  DOutMin=[]  DOutMax=[]  NOutMin=[]  NOutMax=[]  KbOutMin=[]  KbOutMax=[]  KtOutMin=[]  KtOutMax=[]  IntegratorOutMin=[]  IntegratorOutMax=[]  FilterOutMin=[]  FilterOutMax=[]  SumOutMin=[]  SumOutMax=[]  SumI1OutMin=[]  SumI1OutMax=[]  SumI2OutMin=[]  SumI2OutMax=[]  SumI3OutMin=[]  SumI3OutMax=[]  SumDOutMin=[]  SumDOutMax=[]  SaturationOutMin=[]  SaturationOutMax=[]  IntegratorContinuousStateAttributes=''  IntegratorStateMustResolveToSignalObject=off  IntegratorRTWStateStorageClass=Auto  FilterContinuousStateAttributes=''  FilterStateMustResolveToSignalObject=off  FilterRTWStateStorageClass=Auto
  Sum1 : Sum  Inputs=|+-
  W_act : Outport
  wires:
  Load Torque/1 -> PMDC Motor Model/2(Tl)
  W_ref/1 -> Mux/1, Saturation/1
  PMDC Motor Model/1(Theta) -> Right Motor/1
  PMDC Motor Model/3(I) -> Right Motor/3
  Sum1/1 -> Speed PID Controller/1
  PMDC Motor Model/2(w) -> Quantizer/1
  Saturation/1 -> Sum1/1
  Speed PID Controller/1 -> PMDC Motor Model/1(V)
  Mux/1 -> Right Motor Ref vs Act Speed/1
  Quantizer/1 -> W_act/1, Mux/2, Sum1/2, Right Motor/2

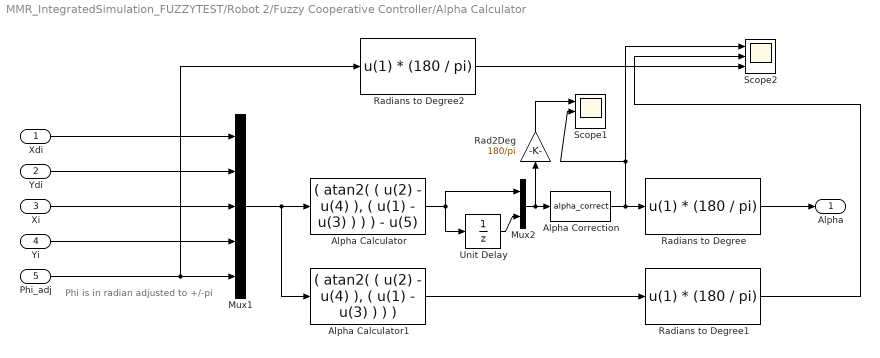
== system MMR_IntegratedSimulation_FUZZYTEST/Robot 2/Fuzzy Cooperative Controller/Alpha Calculator ==
  note: Phi is in radian adjusted to +/-pi
  Xdi : Inport
  Ydi : Inport  Port=2
  Xi : Inport  Port=3
  Yi : Inport  Port=4
  Phi_adj : Inport  Port=5
  Alpha Calculator : Fcn  Expr=( atan2( ( u(2) - u(4) ), ( u(1) - u(3) ) ) ) - u(5)
  Alpha Calculator1 : Fcn  Expr=( atan2( ( u(2) - u(4) ), ( u(1) - u(3) ) ) )
  Alpha Correction : MATLABFcn  MATLABFcn=alpha_correct
  Mux1 : Mux  Inputs=5
  Mux2 : Mux  Inputs=2
  Rad2Deg : Gain  Gain=180/pi
  Radians to Degree : Fcn  Expr=u(1) * (180 / pi)
  Radians to Degree1 : Fcn  Expr=u(1) * (180 / pi)
  Radians to Degree2 : Fcn  Expr=u(1) * (180 / pi)
  Scope1 : Scope  NumInputPorts=3
      settings: YMin=-325~-200~-175  YMax=50~200~200  SaveName=ScopeData4
  Scope2 : Scope  NumInputPorts=3
      settings: YMin=-325~-200~-175  YMax=50~200~200  SaveName=ScopeData2
  Unit Delay : UnitDelay  SampleTime=-1
  Alpha : Outport
  wires:
  Xi/1 -> Mux1/3
  Ydi/1 -> Mux1/2
  Xdi/1 -> Mux1/1
  Mux1/1 -> Alpha Calculator1/1, Alpha Calculator/1
  Yi/1 -> Mux1/4
  Phi_adj/1 -> Mux1/5, Radians to Degree2/1
  Radians to Degree/1 -> Alpha/1
  Alpha Calculator1/1 -> Radians to Degree1/1
  Radians to Degree1/1 -> Scope2/2
  Radians to Degree2/1 -> Scope2/3
  Alpha Correction/1 -> Radians to Degree/1, Scope2/1, Scope1/2
  Mux2/1 -> Alpha Correction/1, Rad2Deg/1
  Alpha Calculator/1 -> Unit Delay/1, Mux2/1
  Unit Delay/1 -> Mux2/2
  Rad2Deg/1 -> Scope1/1

== system MMR_IntegratedSimulation_FUZZYTEST/Robot 2/Fuzzy Cooperative Controller/Drp Calculator ==
  Xdi : Inport
  Ydi : Inport  Port=2
  Xi : Inport  Port=3
  Yi : Inport  Port=4
  Calculate Distance : Fcn  Expr="sqrt( ( u(1) - u(3) )^2 +  ( u(2) - u(4) )^2   )"
  Mux1 : Mux
  Drp : Outport
  wires:
  Mux1/1 -> Calculate Distance/1
  Calculate Distance/1 -> Drp/1
  Xdi/1 -> Mux1/1
  Ydi/1 -> Mux1/2
  Xi/1 -> Mux1/3
  Yi/1 -> Mux1/4

== system MMR_IntegratedSimulation_FUZZYTEST/Robot 2/Fuzzy Cooperative Controller/Phi Calculation ==
  Phi : Inport
  Interpreted MATLAB Function : MATLABFcn  MATLABFcn=PhiAdjust
  Phi_adj : Outport
  wires:
  Phi/1 -> Interpreted MATLAB Function/1
  Interpreted MATLAB Function/1 -> Phi_adj/1

== system MMR_IntegratedSimulation_FUZZYTEST/Robot 2/Fuzzy Cooperative Controller/Xerr Calculator ==
  note: Phi is in radian adjusted to +/-pi
  Xdi : Inport
  Ydi : Inport  Port=2
  Xi : Inport  Port=3
  Yi : Inport  Port=4
  Phi_adj : Inport  Port=5
  Mux1 : Mux  Inputs=5
  Xerr Distance : Fcn  Expr="( cos( u(5) ) * ( u(1) - u(3) ) ) +  ( sin( u(5) ) * ( ( u(2) - u(4) ) ) )"
  Xerr : Outport
  wires:
  Xi/1 -> Mux1/3
  Ydi/1 -> Mux1/2
  Xdi/1 -> Mux1/1
  Xerr Distance/1 -> Xerr/1
  Mux1/1 -> Xerr Distance/1
  Yi/1 -> Mux1/4
  Phi_adj/1 -> Mux1/5

== system MMR_IntegratedSimulation_FUZZYTEST/Robot 2/Fuzzy Cooperative Controller/Yerr Calculator ==
  note: Phi is in radian adjusted to +/-pi
  Xdi : Inport
  Ydi : Inport  Port=2
  Xi : Inport  Port=3
  Yi : Inport  Port=4
  Phi_adj : Inport  Port=5
  Mux1 : Mux  Inputs=5
  Yerr Distance : Fcn  Expr=-( sin( u(5) ) * ( ( u(1) - u(3) ) ) ) + ( cos( u(5) ) * ( u(2) - u(4) ) )
  Yerr : Outport
  wires:
  Phi_adj/1 -> Mux1/5
  Yi/1 -> Mux1/4
  Mux1/1 -> Yerr Distance/1
  Yerr Distance/1 -> Yerr/1
  Xdi/1 -> Mux1/1
  Ydi/1 -> Mux1/2
  Xi/1 -> Mux1/3

== system MMR_IntegratedSimulation_FUZZYTEST/Robot 2/Wheel Motor Controller/Left Motor Speed Controller and Motor Model ==
  W_ref : Inport
  Left Motor Ref vs Act Speed : Scope
      settings: TimeRange=20  YMin=-0.01  YMax=0.12  SaveName=ScopeData6
  Load Torque : Constant  Value=0
  Mux : Mux  Inputs=2
  PMDC Motor Model : Subsystem
  Quantizer : Quantizer  QuantizationInterval=0.001
  Right Motor : Scope  NumInputPorts=3
      settings: TimeRange=20  YMin=-5~-5~-5  YMax=5~5~5
  Saturation : Saturate  UpperLimit=2000  LowerLimit=-2000
  Speed PID Controller : simulink/Continuous/PID Controller  Controller=PID  TimeDomain=Continuous-time  SampleTime=1  IntegratorMethod=Forward Euler  FilterMethod=Forward Euler  Form=Parallel  P=1.39131822817714  I=9.69423314548269  D=-0.0516542631137251  N=13.2920819861493  InitialConditionSource=internal  InitialConditionForIntegrator=0  InitialConditionForFilter=0  ExternalReset=none  LimitOutput=off  UpperSaturationLimit=160  LowerSaturationLimit=-160  LinearizeAsGain=on  AntiWindupMode=none  Kb=1  TrackingMode=off  Kt=1  PParamMin=[]  PParamMax=[]  IParamMin=[]  IParamMax=[]  DParamMin=[]  DParamMax=[]  NParamMin=[]  NParamMax=[]  KbParamMin=[]  KbParamMax=[]  KtParamMin=[]  KtParamMax=[]  POutMin=[]  POutMax=[]  IOutMin=[]  IOutMax=[]  DOutMin=[]  DOutMax=[]  NOutMin=[]  NOutMax=[]  KbOutMin=[]  KbOutMax=[]  KtOutMin=[]  KtOutMax=[]  IntegratorOutMin=[]  IntegratorOutMax=[]  FilterOutMin=[]  FilterOutMax=[]  SumOutMin=[]  SumOutMax=[]  SumI1OutMin=[]  SumI1OutMax=[]  SumI2OutMin=[]  SumI2OutMax=[]  SumI3OutMin=[]  SumI3OutMax=[]  SumDOutMin=[]  SumDOutMax=[]  SaturationOutMin=[]  SaturationOutMax=[]  IntegratorContinuousStateAttributes=''  IntegratorStateMustResolveToSignalObject=off  IntegratorRTWStateStorageClass=Auto  FilterContinuousStateAttributes=''  FilterStateMustResolveToSignalObject=off  FilterRTWStateStorageClass=Auto
  Sum1 : Sum  Inputs=|+-
  W_act : Outport
  wires:
  Speed PID Controller/1 -> PMDC Motor Model/1(V)
  Saturation/1 -> Sum1/1
  PMDC Motor Model/2(w) -> Quantizer/1
  Sum1/1 -> Speed PID Controller/1
  PMDC Motor Model/3(I) -> Right Motor/3
  PMDC Motor Model/1(Theta) -> Right Motor/1
  W_ref/1 -> Mux/1, Saturation/1
  Load Torque/1 -> PMDC Motor Model/2(Tl)
  Mux/1 -> Left Motor Ref vs Act Speed/1
  Quantizer/1 -> W_act/1, Mux/2, Sum1/2, Right Motor/2

== system MMR_IntegratedSimulation_FUZZYTEST/Robot 2/Wheel Motor Controller/Right Motor Speed Controller and Motor Model ==
  W_ref : Inport
  Load Torque : Constant  Value=0
  Mux : Mux  Inputs=2
  PMDC Motor Model : Subsystem
  Quantizer : Quantizer  QuantizationInterval=0.001
  Right Motor : Scope  NumInputPorts=3
      settings: TimeRange=20  YMin=-5~-5~-5  YMax=5~5~5
  Right Motor Ref vs Act Speed : Scope
      settings: TimeRange=20  YMin=-0.01  YMax=0.12
  Saturation : Saturate  UpperLimit=2000  LowerLimit=-2000
  Speed PID Controller : simulink/Continuous/PID Controller  Controller=PID  TimeDomain=Continuous-time  SampleTime=1  IntegratorMethod=Forward Euler  FilterMethod=Forward Euler  Form=Parallel  P=1.39131822817714  I=9.69423314548269  D=-0.0516542631137251  N=13.2920819861493  InitialConditionSource=internal  InitialConditionForIntegrator=0  InitialConditionForFilter=0  ExternalReset=none  LimitOutput=off  UpperSaturationLimit=160  LowerSaturationLimit=-160  LinearizeAsGain=on  AntiWindupMode=none  Kb=1  TrackingMode=off  Kt=1  PParamMin=[]  PParamMax=[]  IParamMin=[]  IParamMax=[]  DParamMin=[]  DParamMax=[]  NParamMin=[]  NParamMax=[]  KbParamMin=[]  KbParamMax=[]  KtParamMin=[]  KtParamMax=[]  POutMin=[]  POutMax=[]  IOutMin=[]  IOutMax=[]  DOutMin=[]  DOutMax=[]  NOutMin=[]  NOutMax=[]  KbOutMin=[]  KbOutMax=[]  KtOutMin=[]  KtOutMax=[]  IntegratorOutMin=[]  IntegratorOutMax=[]  FilterOutMin=[]  FilterOutMax=[]  SumOutMin=[]  SumOutMax=[]  SumI1OutMin=[]  SumI1OutMax=[]  SumI2OutMin=[]  SumI2OutMax=[]  SumI3OutMin=[]  SumI3OutMax=[]  SumDOutMin=[]  SumDOutMax=[]  SaturationOutMin=[]  SaturationOutMax=[]  IntegratorContinuousStateAttributes=''  IntegratorStateMustResolveToSignalObject=off  IntegratorRTWStateStorageClass=Auto  FilterContinuousStateAttributes=''  FilterStateMustResolveToSignalObject=off  FilterRTWStateStorageClass=Auto
  Sum1 : Sum  Inputs=|+-
  W_act : Outport
  wires:
  Load Torque/1 -> PMDC Motor Model/2(Tl)
  W_ref/1 -> Mux/1, Saturation/1
  PMDC Motor Model/1(Theta) -> Right Motor/1
  PMDC Motor Model/3(I) -> Right Motor/3
  Sum1/1 -> Speed PID Controller/1
  PMDC Motor Model/2(w) -> Quantizer/1
  Saturation/1 -> Sum1/1
  Speed PID Controller/1 -> PMDC Motor Model/1(V)
  Mux/1 -> Right Motor Ref vs Act Speed/1
  Quantizer/1 -> W_act/1, Mux/2, Sum1/2, Right Motor/2

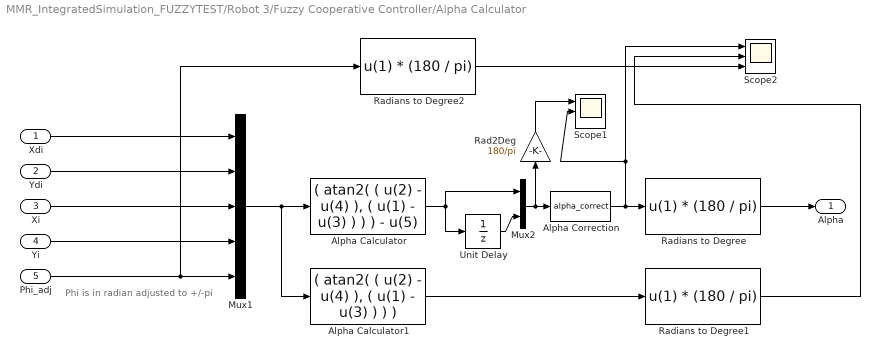
== system MMR_IntegratedSimulation_FUZZYTEST/Robot 3/Fuzzy Cooperative Controller/Alpha Calculator ==
  note: Phi is in radian adjusted to +/-pi
  Xdi : Inport
  Ydi : Inport  Port=2
  Xi : Inport  Port=3
  Yi : Inport  Port=4
  Phi_adj : Inport  Port=5
  Alpha Calculator : Fcn  Expr=( atan2( ( u(2) - u(4) ), ( u(1) - u(3) ) ) ) - u(5)
  Alpha Calculator1 : Fcn  Expr=( atan2( ( u(2) - u(4) ), ( u(1) - u(3) ) ) )
  Alpha Correction : MATLABFcn  MATLABFcn=alpha_correct
  Mux1 : Mux  Inputs=5
  Mux2 : Mux  Inputs=2
  Rad2Deg : Gain  Gain=180/pi
  Radians to Degree : Fcn  Expr=u(1) * (180 / pi)
  Radians to Degree1 : Fcn  Expr=u(1) * (180 / pi)
  Radians to Degree2 : Fcn  Expr=u(1) * (180 / pi)
  Scope1 : Scope  NumInputPorts=3
      settings: YMin=-325~-200~-175  YMax=50~200~200  SaveName=ScopeData4
  Scope2 : Scope  NumInputPorts=3
      settings: YMin=-325~-200~-175  YMax=50~200~200  SaveName=ScopeData2
  Unit Delay : UnitDelay  SampleTime=-1
  Alpha : Outport
  wires:
  Xi/1 -> Mux1/3
  Ydi/1 -> Mux1/2
  Xdi/1 -> Mux1/1
  Mux1/1 -> Alpha Calculator1/1, Alpha Calculator/1
  Yi/1 -> Mux1/4
  Phi_adj/1 -> Mux1/5, Radians to Degree2/1
  Radians to Degree/1 -> Alpha/1
  Alpha Calculator1/1 -> Radians to Degree1/1
  Radians to Degree1/1 -> Scope2/2
  Radians to Degree2/1 -> Scope2/3
  Alpha Correction/1 -> Radians to Degree/1, Scope2/1, Scope1/2
  Mux2/1 -> Alpha Correction/1, Rad2Deg/1
  Alpha Calculator/1 -> Unit Delay/1, Mux2/1
  Unit Delay/1 -> Mux2/2
  Rad2Deg/1 -> Scope1/1

== system MMR_IntegratedSimulation_FUZZYTEST/Robot 3/Fuzzy Cooperative Controller/Drp Calculator ==
  Xdi : Inport
  Ydi : Inport  Port=2
  Xi : Inport  Port=3
  Yi : Inport  Port=4
  Calculate Distance : Fcn  Expr="sqrt( ( u(1) - u(3) )^2 +  ( u(2) - u(4) )^2   )"
  Mux1 : Mux
  Drp : Outport
  wires:
  Mux1/1 -> Calculate Distance/1
  Calculate Distance/1 -> Drp/1
  Xdi/1 -> Mux1/1
  Ydi/1 -> Mux1/2
  Xi/1 -> Mux1/3
  Yi/1 -> Mux1/4

== system MMR_IntegratedSimulation_FUZZYTEST/Robot 3/Fuzzy Cooperative Controller/Phi Calculation ==
  Phi : Inport
  Interpreted MATLAB Function : MATLABFcn  MATLABFcn=PhiAdjust
  Phi_adj : Outport
  wires:
  Phi/1 -> Interpreted MATLAB Function/1
  Interpreted MATLAB Function/1 -> Phi_adj/1

== system MMR_IntegratedSimulation_FUZZYTEST/Robot 3/Fuzzy Cooperative Controller/Xerr Calculator ==
  note: Phi is in radian adjusted to +/-pi
  Xdi : Inport
  Ydi : Inport  Port=2
  Xi : Inport  Port=3
  Yi : Inport  Port=4
  Phi_adj : Inport  Port=5
  Mux1 : Mux  Inputs=5
  Xerr Distance : Fcn  Expr="( cos( u(5) ) * ( u(1) - u(3) ) ) +  ( sin( u(5) ) * ( ( u(2) - u(4) ) ) )"
  Xerr : Outport
  wires:
  Xi/1 -> Mux1/3
  Ydi/1 -> Mux1/2
  Xdi/1 -> Mux1/1
  Xerr Distance/1 -> Xerr/1
  Mux1/1 -> Xerr Distance/1
  Yi/1 -> Mux1/4
  Phi_adj/1 -> Mux1/5

== system MMR_IntegratedSimulation_FUZZYTEST/Robot 3/Fuzzy Cooperative Controller/Yerr Calculator ==
  note: Phi is in radian adjusted to +/-pi
  Xdi : Inport
  Ydi : Inport  Port=2
  Xi : Inport  Port=3
  Yi : Inport  Port=4
  Phi_adj : Inport  Port=5
  Mux1 : Mux  Inputs=5
  Yerr Distance : Fcn  Expr=-( sin( u(5) ) * ( ( u(1) - u(3) ) ) ) + ( cos( u(5) ) * ( u(2) - u(4) ) )
  Yerr : Outport
  wires:
  Phi_adj/1 -> Mux1/5
  Yi/1 -> Mux1/4
  Mux1/1 -> Yerr Distance/1
  Yerr Distance/1 -> Yerr/1
  Xdi/1 -> Mux1/1
  Ydi/1 -> Mux1/2
  Xi/1 -> Mux1/3

== system MMR_IntegratedSimulation_FUZZYTEST/Robot 3/Wheel Motor Controller/Left Motor Speed Controller and Motor Model ==
  W_ref : Inport
  Left Motor Ref vs Act Speed : Scope
      settings: TimeRange=20  YMin=-0.01  YMax=0.12  SaveName=ScopeData6
  Load Torque : Constant  Value=0
  Mux : Mux  Inputs=2
  PMDC Motor Model : Subsystem
  Quantizer : Quantizer  QuantizationInterval=0.001
  Right Motor : Scope  NumInputPorts=3
      settings: TimeRange=20  YMin=-5~-5~-5  YMax=5~5~5
  Saturation : Saturate  UpperLimit=2000  LowerLimit=-2000
  Speed PID Controller : simulink/Continuous/PID Controller  Controller=PID  TimeDomain=Continuous-time  SampleTime=1  IntegratorMethod=Forward Euler  FilterMethod=Forward Euler  Form=Parallel  P=1.39131822817714  I=9.69423314548269  D=-0.0516542631137251  N=13.2920819861493  InitialConditionSource=internal  InitialConditionForIntegrator=0  InitialConditionForFilter=0  ExternalReset=none  LimitOutput=off  UpperSaturationLimit=160  LowerSaturationLimit=-160  LinearizeAsGain=on  AntiWindupMode=none  Kb=1  TrackingMode=off  Kt=1  PParamMin=[]  PParamMax=[]  IParamMin=[]  IParamMax=[]  DParamMin=[]  DParamMax=[]  NParamMin=[]  NParamMax=[]  KbParamMin=[]  KbParamMax=[]  KtParamMin=[]  KtParamMax=[]  POutMin=[]  POutMax=[]  IOutMin=[]  IOutMax=[]  DOutMin=[]  DOutMax=[]  NOutMin=[]  NOutMax=[]  KbOutMin=[]  KbOutMax=[]  KtOutMin=[]  KtOutMax=[]  IntegratorOutMin=[]  IntegratorOutMax=[]  FilterOutMin=[]  FilterOutMax=[]  SumOutMin=[]  SumOutMax=[]  SumI1OutMin=[]  SumI1OutMax=[]  SumI2OutMin=[]  SumI2OutMax=[]  SumI3OutMin=[]  SumI3OutMax=[]  SumDOutMin=[]  SumDOutMax=[]  SaturationOutMin=[]  SaturationOutMax=[]  IntegratorContinuousStateAttributes=''  IntegratorStateMustResolveToSignalObject=off  IntegratorRTWStateStorageClass=Auto  FilterContinuousStateAttributes=''  FilterStateMustResolveToSignalObject=off  FilterRTWStateStorageClass=Auto
  Sum1 : Sum  Inputs=|+-
  W_act : Outport
  wires:
  Speed PID Controller/1 -> PMDC Motor Model/1(V)
  Saturation/1 -> Sum1/1
  PMDC Motor Model/2(w) -> Quantizer/1
  Sum1/1 -> Speed PID Controller/1
  PMDC Motor Model/3(I) -> Right Motor/3
  PMDC Motor Model/1(Theta) -> Right Motor/1
  W_ref/1 -> Mux/1, Saturation/1
  Load Torque/1 -> PMDC Motor Model/2(Tl)
  Mux/1 -> Left Motor Ref vs Act Speed/1
  Quantizer/1 -> W_act/1, Mux/2, Sum1/2, Right Motor/2

== system MMR_IntegratedSimulation_FUZZYTEST/Robot 3/Wheel Motor Controller/Right Motor Speed Controller and Motor Model ==
  W_ref : Inport
  Load Torque : Constant  Value=0
  Mux : Mux  Inputs=2
  PMDC Motor Model : Subsystem
  Quantizer : Quantizer  QuantizationInterval=0.001
  Right Motor : Scope  NumInputPorts=3
      settings: TimeRange=20  YMin=-5~-5~-5  YMax=5~5~5
  Right Motor Ref vs Act Speed : Scope
      settings: TimeRange=20  YMin=-0.01  YMax=0.12
  Saturation : Saturate  UpperLimit=2000  LowerLimit=-2000
  Speed PID Controller : simulink/Continuous/PID Controller  Controller=PID  TimeDomain=Continuous-time  SampleTime=1  IntegratorMethod=Forward Euler  FilterMethod=Forward Euler  Form=Parallel  P=1.39131822817714  I=9.69423314548269  D=-0.0516542631137251  N=13.2920819861493  InitialConditionSource=internal  InitialConditionForIntegrator=0  InitialConditionForFilter=0  ExternalReset=none  LimitOutput=off  UpperSaturationLimit=160  LowerSaturationLimit=-160  LinearizeAsGain=on  AntiWindupMode=none  Kb=1  TrackingMode=off  Kt=1  PParamMin=[]  PParamMax=[]  IParamMin=[]  IParamMax=[]  DParamMin=[]  DParamMax=[]  NParamMin=[]  NParamMax=[]  KbParamMin=[]  KbParamMax=[]  KtParamMin=[]  KtParamMax=[]  POutMin=[]  POutMax=[]  IOutMin=[]  IOutMax=[]  DOutMin=[]  DOutMax=[]  NOutMin=[]  NOutMax=[]  KbOutMin=[]  KbOutMax=[]  KtOutMin=[]  KtOutMax=[]  IntegratorOutMin=[]  IntegratorOutMax=[]  FilterOutMin=[]  FilterOutMax=[]  SumOutMin=[]  SumOutMax=[]  SumI1OutMin=[]  SumI1OutMax=[]  SumI2OutMin=[]  SumI2OutMax=[]  SumI3OutMin=[]  SumI3OutMax=[]  SumDOutMin=[]  SumDOutMax=[]  SaturationOutMin=[]  SaturationOutMax=[]  IntegratorContinuousStateAttributes=''  IntegratorStateMustResolveToSignalObject=off  IntegratorRTWStateStorageClass=Auto  FilterContinuousStateAttributes=''  FilterStateMustResolveToSignalObject=off  FilterRTWStateStorageClass=Auto
  Sum1 : Sum  Inputs=|+-
  W_act : Outport
  wires:
  Load Torque/1 -> PMDC Motor Model/2(Tl)
  W_ref/1 -> Mux/1, Saturation/1
  PMDC Motor Model/1(Theta) -> Right Motor/1
  PMDC Motor Model/3(I) -> Right Motor/3
  Sum1/1 -> Speed PID Controller/1
  PMDC Motor Model/2(w) -> Quantizer/1
  Saturation/1 -> Sum1/1
  Speed PID Controller/1 -> PMDC Motor Model/1(V)
  Mux/1 -> Right Motor Ref vs Act Speed/1
  Quantizer/1 -> W_act/1, Mux/2, Sum1/2, Right Motor/2

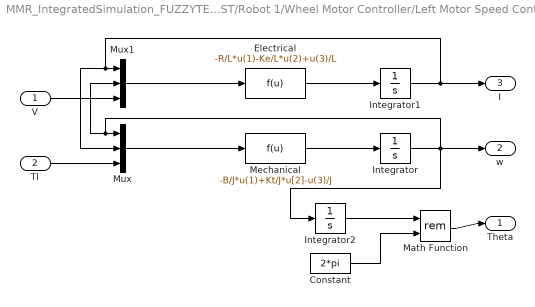
== system MMR_IntegratedSimulation_FUZZYTEST/Robot 1/Wheel Motor Controller/Left Motor Speed Controller and Motor Model/PMDC Motor Model ==
  V : Inport
  Tl : Inport  Port=2
  Constant : Constant  Value=2*pi
  Electrical : Fcn  Expr=-R/L*u(1)-Ke/L*u(2)+u(3)/L
  Integrator : Integrator
  Integrator1 : Integrator
  Integrator2 : Integrator
  Math Function : Math  Operator=rem  SaturateOnIntegerOverflow=on
  Mechanical : Fcn  Expr=-B/J*u(1)+Kt/J*u[2]-u(3)/J
  Mux : Mux  Inputs=3
  Mux1 : Mux  Inputs=3
  Theta : Outport
  w : Outport  Port=2
  I : Outport  Port=3
  wires:
  Constant/1 -> Math Function/2
  Integrator2/1 -> Math Function/1
  Math Function/1 -> Theta/1
  V/1 -> Mux1/3
  Integrator/1 -> Integrator2/1, Mux/1, Mux1/2, w/1
  Mux1/1 -> Electrical/1
  Electrical/1 -> Integrator1/1
  Integrator1/1 -> Mux/2, Mux1/1, I/1
  Mechanical/1 -> Integrator/1
  Tl/1 -> Mux/3
  Mux/1 -> Mechanical/1

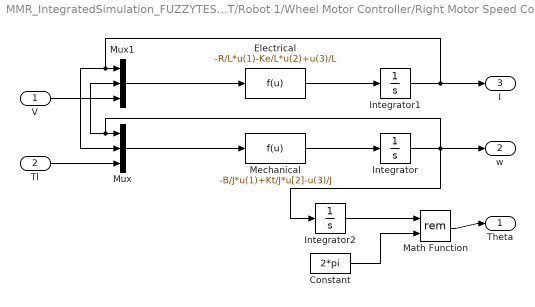
== system MMR_IntegratedSimulation_FUZZYTEST/Robot 1/Wheel Motor Controller/Right Motor Speed Controller and Motor Model/PMDC Motor Model ==
  V : Inport
  Tl : Inport  Port=2
  Constant : Constant  Value=2*pi
  Electrical : Fcn  Expr=-R/L*u(1)-Ke/L*u(2)+u(3)/L
  Integrator : Integrator
  Integrator1 : Integrator
  Integrator2 : Integrator
  Math Function : Math  Operator=rem  SaturateOnIntegerOverflow=on
  Mechanical : Fcn  Expr=-B/J*u(1)+Kt/J*u[2]-u(3)/J
  Mux : Mux  Inputs=3
  Mux1 : Mux  Inputs=3
  Theta : Outport
  w : Outport  Port=2
  I : Outport  Port=3
  wires:
  Mux/1 -> Mechanical/1
  Tl/1 -> Mux/3
  Mechanical/1 -> Integrator/1
  Integrator1/1 -> I/1, Mux1/1, Mux/2
  Electrical/1 -> Integrator1/1
  Mux1/1 -> Electrical/1
  Integrator/1 -> w/1, Mux1/2, Mux/1, Integrator2/1
  V/1 -> Mux1/3
  Math Function/1 -> Theta/1
  Integrator2/1 -> Math Function/1
  Constant/1 -> Math Function/2
